simulink model "part2"  (R2020b)
settings: Solver=FixedStepDiscrete  StartTime=0.0  StopTime=10  RelTol=1e-3
settings Model: Creator=superdeano  LastModifiedBy=superdeano

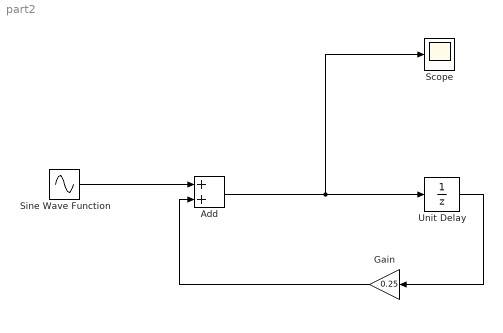
== system part2 ==
  Add : Sum
  Gain : Gain  Gain=0.25
  Scope : Scope
  Sine Wave Function : Sin  SineType=Sample based  Frequency=2* pi * (1/150)  SampleTime=0.1
  Unit Delay : UnitDelay  SampleTime=-1  HasFrameUpgradeWarning=on
  wires:
  Sine Wave Function/1 -> Add/1
  Gain/1 -> Add/2
  Add/1 -> Scope/1, Unit Delay/1
  Unit Delay/1 -> Gain/1
